simulink model "FCC"  (R2018b)
settings: Solver=FixedStepDiscrete  StartTime=0.0  StopTime=10.0  FixedStep=0.001  RelTol=1e-3  EnableMultiTasking=on
undefined symbols (not defined in the file): Kd, Ki, Kp
libraries: simulink x1
Description:
  | This model represents a flight control system for a helicopter that controls pitch attitude, roll attitude and yaw rate based on pilot inputs from the cyclic and pedals. The flight control computer also closes the loop on three hydrualic actuators and has sensor inputs from three Attitude/Heading Reference Systems.
settings Model: Creator=bpotter  LastModifiedBy=bpotter
settings DataIOCC: LimitDataPoints=on
settings OptimizationCC: BlockReduction=off  DefaultParameterBehavior=Inlined  UseDivisionForNetSlopeComputation=on  InitFltsAndDblsToZero=on  EfficientFloat2IntCast=on  EfficientMapNaN2IntZero=off  LifeSpan=inf  MaxStackSize=inf
settings DebuggingCC: SignalInfNanChecking=error  SignalRangeChecking=error  ReadBeforeWriteMsg=EnableAllAsError  WriteAfterWriteMsg=EnableAllAsError  WriteAfterReadMsg=EnableAllAsError  AlgebraicLoopMsg=error  ArtificialAlgebraicLoopMsg=error  SaveWithDisabledLinksMsg=error  SaveWithParameterizedLinksMsg=error  BlockPriorityViolationMsg=error  SolverPrmCheckMsg=error  InheritedTsInSrcMsg=error  SingleTaskRateTransMsg=error  TasksWithSamePriorityMsg=error  SigSpecEnsureSampleTimeMsg=error  CheckMatrixSingularityMsg=error  IntegerOverflowMsg=error  ParameterUnderflowMsg=error  ParameterPrecisionLossMsg=error  ParameterTunabilityLossMsg=error  UnderSpecifiedDataTypeMsg=error  UnnecessaryDatatypeConvMsg=warning  VectorMatrixConversionMsg=error  SignalLabelMismatchMsg=error  UnconnectedInputMsg=error  UnconnectedOutputMsg=error  UnconnectedLineMsg=error  SFcnCompatibilityMsg=error  UniqueDataStoreMsg=error  BusObjectLabelMismatch=error  RootOutportRequireBusObject=error  AssertControl=DisableAll  AllowSymbolicDim=off  ModelReferenceIOMsg=error  ModelReferenceIOMismatchMessage=error  UnknownTsInhSupMsg=error  ModelReferenceDataLoggingMessage=error  StateNameClashWarn=warning  LibraryContextMissingDiagnostic=none  StrictBusMsg=ErrorOnBusTreatedAsVector  NonBusSignalsTreatedAsBus=error  SFInvalidInputDataAccessInChartInitDiag=error  SFTransitionOutsideNaturalParentDiag=error  SFUnreachableExecutionPathDiag=error  SFUndirectedBroadcastEventsDiag=error  SFTransitionActionBeforeConditionDiag=error  SFExecutionAtInitializationDiag=none  IntegerSaturationMsg=error
settings HardwareCC: ProdBitPerPointer=32  ProdBitPerSizeT=32  ProdBitPerPtrDiffT=32  ProdWordSize=32  ProdHWDeviceType=Intel->x86-32 (Windows32)  TargetIntDivRoundTo=Zero
settings ModelReferenceCC: PropagateSignalLabelsOutOfModel=off
settings SFSimCC: SimUseLocalCustomCode=off  CompileTimeRecursionLimit=0  EnableRuntimeRecursion=off  MATLABDynamicMemAlloc=off
settings RTWCC: SystemTargetFile=ert.tlc  TemplateMakefile=ert_default_tmf  GenerateReport=on  RTWUseLocalCustomCode=off  IncludeHyperlinkInReport=on  LaunchReport=on  PortableWordSizes=on  GenerateTraceInfo=on  GenerateTraceReport=on  GenerateTraceReportSl=on  GenerateTraceReportSf=on  GenerateTraceReportEml=on
settings CodeAppCC: ForceParamTrailComments=on  IgnoreCustomStorageClasses=off  MangleLength=4  StateflowObjectComments=on  ReqsInCode=on
settings ERTTargetCC: TargetLangStandard=C99 (ISO)  UtilityFuncGeneration=Shared location  MultiwordLength=2048  GenerateSampleERTMain=on  IncludeMdlTerminateFcn=off  SuppressErrorStatus=on  SupportAbsoluteTime=off  SupportNonFinite=off  ParenthesesLevel=Maximum  CastingMode=Standards  GenerateSharedConstants=off  ERTCustomFileTemplate=example_file_process.tlc  ERTFilePackagingFormat=Compact  PreserveExpressionOrder=on  PreserveIfCondition=on  ConvertIfToSwitch=off  SuppressUnreachableDefaultCases=off  EnableSignedLeftShifts=off  EnableSignedRightShifts=off
settings ConfigComp: CovMetricSettings=dw  CovHtmlReporting=on  CovSaveCumulativeToWorkspaceVar=on  CovSaveSingleToWorkspaceVar=on  CovExternalEMLEnable=off  CovSFcnEnable=off  PSOpenProjectManager=on  PSResultDir=CodeProver_results_$ModelName$  PSModelRefVerifDepth=All  PSAutoStubLUT=off  DVTestSuiteOptimization=CombinedObjectives (Nonlinear Extended)  DVDetectOutOfBounds=on  DVDesignMinMaxCheck=on

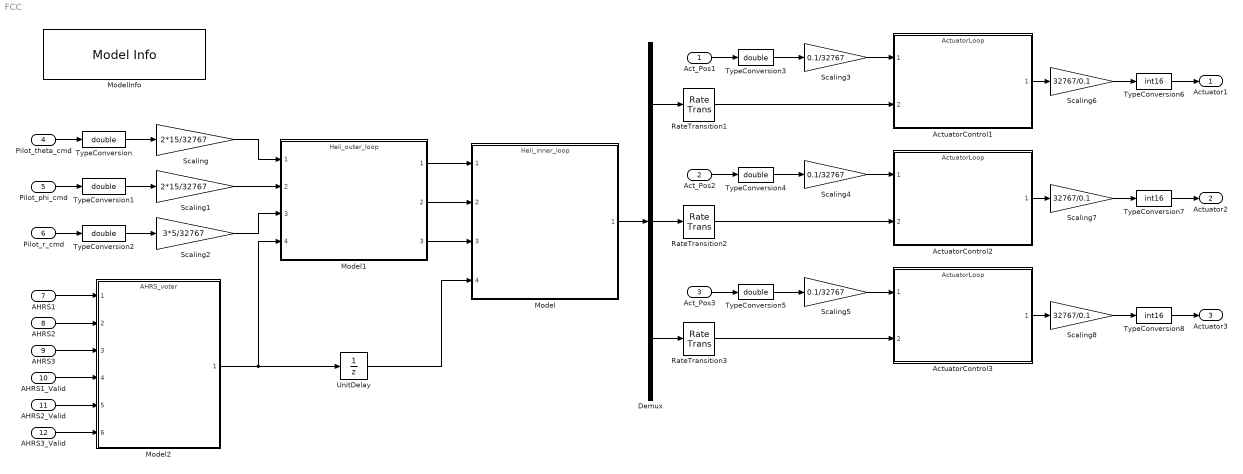
== system FCC ==
  Act_Pos1 : Inport  RequirementInfo={} %GIDa_bd07c6dd_f370_4b97_930d_e4b4981f6696  OutMin=-32768  OutMax=32767  OutDataTypeStr=int16  PortDimensions=1  SampleTime=0.001
  Act_Pos2 : Inport  RequirementInfo={} %GIDa_befe8f2a_df1a_408c_ad43_982e86d61679  Port=2  OutMin=-32768  OutMax=32767  OutDataTypeStr=int16  PortDimensions=1  SampleTime=0.001
  Act_Pos3 : Inport  RequirementInfo={} %GIDa_31a40888_6c46_41b4_95a0_85353469c339  Port=3  OutMin=-32768  OutMax=32767  OutDataTypeStr=int16  PortDimensions=1  SampleTime=0.001
  Pilot_theta_cmd : Inport  RequirementInfo={} %GIDa_db7610c8_fc0b_436a_9176_d063f912f7d4  Port=4  OutMin=-32768  OutMax=32767  OutDataTypeStr=int16  PortDimensions=1  SampleTime=0.01
  Pilot_phi_cmd : Inport  RequirementInfo={} %GIDa_c88793d4_8072_44c9_b7b8_fa9c7a9d095b  Port=5  OutMin=-32768  OutMax=32767  OutDataTypeStr=int16  PortDimensions=1  SampleTime=0.01
  Pilot_r_cmd : Inport  RequirementInfo={} %GIDa_dcbca35e_d37f_4666_ab6e_90461c32e72b  Port=6  OutMin=-32768  OutMax=32767  OutDataTypeStr=int16  PortDimensions=1  SampleTime=0.01
  AHRS1 : Inport  RequirementInfo={} %GIDa_80750aa2_e003_442f_b031_591405abb5b4  Port=7  OutMin=-180  OutMax=180  OutDataTypeStr=double  PortDimensions=5  SampleTime=0.01
  AHRS2 : Inport  RequirementInfo={} %GIDa_426ecfe9_991d_4f5f_80a1_3ebd9c43cb2d  Port=8  OutMin=-180  OutMax=180  OutDataTypeStr=double  PortDimensions=5  SampleTime=0.01
  AHRS3 : Inport  RequirementInfo={} %GIDa_78c653e8_6a57_498e_82a6_5c1330482b46  Port=9  OutMin=-180  OutMax=180  OutDataTypeStr=double  PortDimensions=5  SampleTime=0.01
  AHRS1_Valid : Inport  RequirementInfo={} %GIDa_98b30cb9_b983_4ea0_884e_7d00cc40e0ae  Port=10  OutMin=0  OutMax=1  OutDataTypeStr=boolean  PortDimensions=1  SampleTime=0.01
  AHRS2_Valid : Inport  RequirementInfo={} %GIDa_97bebaab_bb97_4960_9c93_3ab597d65b2c  Port=11  OutMin=0  OutMax=1  OutDataTypeStr=boolean  PortDimensions=1  SampleTime=0.01
  AHRS3_Valid : Inport  RequirementInfo={} %GIDa_19fd269e_922e_4b90_a0a1_f582c1a1233f  Port=12  OutMin=0  OutMax=1  OutDataTypeStr=boolean  PortDimensions=1  SampleTime=0.01
  ActuatorControl1 : ModelReference  RequirementInfo={} %GIDa_286e3d14_20d8_4bab_aa60_69e0b735c692  ModelNameDialog=ActuatorLoop  ParameterArgumentNames=Kp,Kd,Ki  ParameterArgumentValues=0.3,0.02,0.12  UsingDefaultArgumentValue=0,0,0  SimulationMode=Normal  ModelReferenceVersion=1.40
  ActuatorControl2 : ModelReference  RequirementInfo={} %GIDa_6f1d74b9_a492_4876_bea7_840580edc6b2  ModelNameDialog=ActuatorLoop  ParameterArgumentNames=Kp,Kd,Ki  ParameterArgumentValues=0.3,0.02,0.12  UsingDefaultArgumentValue=0,0,0  SimulationMode=Normal  ModelReferenceVersion=1.40
  ActuatorControl3 : ModelReference  RequirementInfo={} %GIDa_5780c5a5_fbb9_4ac7_8106_2a6374d1c9b6  ModelNameDialog=ActuatorLoop  ParameterArgumentNames=Kp,Kd,Ki  ParameterArgumentValues=0.3,0.02,0.12  UsingDefaultArgumentValue=0,0,0  SimulationMode=Normal  ModelReferenceVersion=1.40
  Demux : Demux  Outputs=3
  Model : ModelReference  RequirementInfo={} %GIDa_9f86ca98_8be5_4c76_b7e2_fad36800e068  ModelNameDialog=Heli_inner_loop  SimulationMode=Normal  ModelReferenceVersion=1.29
  Model1 : ModelReference  RequirementInfo={} %GIDa_9b6918d6_c850_456e_b2c9_5fe3f7942cab  ModelNameDialog=Heli_outer_loop  SimulationMode=Normal  ModelReferenceVersion=1.27
  Model2 : ModelReference  RequirementInfo={} %GIDa_45ae46d8_e7b6_4c79_9f98_fde151ca045a  ModelNameDialog=AHRS_voter  SimulationMode=Normal  ModelReferenceVersion=1.56
  ModelInfo : simulink/Model-Wide Utilities/Model Info  Frame=on  DisplayStringWithTags=|  HorizontalTextAlignment=Center  LeftAlignmentValue=0.5
      | Model Name: %<ModelName>
      | Model Version: %<ModelVersion>
      | Last Modified: %<LastModificationDate>
      | 
      | Copyright 2016 The MathWorks, Inc.
  RateTransition1 : RateTransition  OutPortSampleTime=0.001
  RateTransition2 : RateTransition  OutPortSampleTime=0.001
  RateTransition3 : RateTransition  OutPortSampleTime=0.001
  Scaling : Gain  RequirementInfo={} %GIDa_1ef55a73_43a4_45d8_95fb_e076cecdcdfb  Gain=2*15/32767
  Scaling1 : Gain  RequirementInfo={} %GIDa_7c0c4402_eed7_48e8_afe7_4e3c25c20a7a  Gain=2*15/32767
  Scaling2 : Gain  RequirementInfo={} %GIDa_c573d4b7_5d38_46e9_91de_b74deab4371c  Gain=3*5/32767
  Scaling3 : Gain  RequirementInfo={} %GIDa_7165c314_723d_4c07_8145_b8a5caf68d15  Gain=0.1/32767
  Scaling4 : Gain  RequirementInfo={} %GIDa_e7d939dc_4756_4c7f_b09b_37bf3b41d91a  Gain=0.1/32767
  Scaling5 : Gain  RequirementInfo={} %GIDa_feb82ae6_ad6e_4307_be71_c8336adce306  Gain=0.1/32767
  Scaling6 : Gain  RequirementInfo={} %GIDa_7472457d_0776_496d_982d_888a9d0ccd31  Gain=32767/0.1  SaturateOnIntegerOverflow=on  OutDataTypeStr=Inherit: Same as input
  Scaling7 : Gain  RequirementInfo={} %GIDa_27270bf9_988e_4404_bcbc_b8b952500a10  Gain=32767/0.1  SaturateOnIntegerOverflow=on  OutDataTypeStr=Inherit: Same as input
  Scaling8 : Gain  RequirementInfo={} %GIDa_610bafad_081e_4b34_b128_56987096ac68  Gain=32767/0.1  SaturateOnIntegerOverflow=on  OutDataTypeStr=Inherit: Same as input
  TypeConversion : DataTypeConversion  RequirementInfo={} %GIDa_507dfc48_2783_4f54_bcc8_b8696a72db7e  OutDataTypeStr=double
  TypeConversion1 : DataTypeConversion  RequirementInfo={} %GIDa_a28ee961_0826_464b_952a_7525a850e69d  OutDataTypeStr=double
  TypeConversion2 : DataTypeConversion  RequirementInfo={} %GIDa_fd029ccd_092a_44ae_ba63_7ba73a38dd29  OutDataTypeStr=double
  TypeConversion3 : DataTypeConversion  RequirementInfo={} %GIDa_1949c14f_f47a_4a2c_b83b_c5a889847ffe  OutDataTypeStr=double
  TypeConversion4 : DataTypeConversion  RequirementInfo={} %GIDa_29dd9675_a919_4bb5_a5f8_82f3a5941f34  OutDataTypeStr=double
  TypeConversion5 : DataTypeConversion  RequirementInfo={} %GIDa_0de29fa2_9bc9_4717_a2b2_9bc25147b395  OutDataTypeStr=double
  TypeConversion6 : DataTypeConversion  RequirementInfo={} %GIDa_6ab4c5ff_fe2f_4ca3_924f_fd1b53f5822d  OutDataTypeStr=int16
  TypeConversion7 : DataTypeConversion  RequirementInfo={} %GIDa_fe351f61_f1d0_4404_aa3c_5114a8d4af07  OutDataTypeStr=int16
  TypeConversion8 : DataTypeConversion  RequirementInfo={} %GIDa_5d4fc6d9_c4e4_4413_b6aa_2af104ad7bd2  OutDataTypeStr=int16
  UnitDelay : UnitDelay  SampleTime=-1
  Actuator1 : Outport  RequirementInfo={} %GIDa_0e27a381_736b_4604_a443_1ce3b6bc89bb
  Actuator2 : Outport  RequirementInfo={} %GIDa_ad165c3e_4ab6_4671_aa0b_225d448592bb  Port=2
  Actuator3 : Outport  RequirementInfo={} %GIDa_f2f33165_edb5_46cb_9250_52960ae67539  Port=3
  wires:
  ActuatorControl1/1 -> Scaling6/1
  ActuatorControl2/1 -> Scaling7/1
  ActuatorControl3/1 -> Scaling8/1
  RateTransition1/1 -> ActuatorControl1/2
  RateTransition2/1 -> ActuatorControl2/2
  RateTransition3/1 -> ActuatorControl3/2
  AHRS2/1 -> Model2/2
  AHRS3/1 -> Model2/3
  Demux/1 -> RateTransition1/1
  Demux/2 -> RateTransition2/1
  Demux/3 -> RateTransition3/1
  Model/1 -> Demux/1
  Model1/1 -> Model/1
  Model1/2 -> Model/2
  Model1/3 -> Model/3
  AHRS1/1 -> Model2/1
  Model2/1 -> Model1/4, UnitDelay/1
  AHRS1_Valid/1 -> Model2/4
  AHRS2_Valid/1 -> Model2/5
  AHRS3_Valid/1 -> Model2/6
  TypeConversion/1 -> Scaling/1
  Pilot_theta_cmd/1 -> TypeConversion/1
  Scaling/1 -> Model1/1
  TypeConversion1/1 -> Scaling1/1
  Pilot_phi_cmd/1 -> TypeConversion1/1
  Scaling1/1 -> Model1/2
  Pilot_r_cmd/1 -> TypeConversion2/1
  TypeConversion2/1 -> Scaling2/1
  Scaling2/1 -> Model1/3
  TypeConversion3/1 -> Scaling3/1
  Act_Pos1/1 -> TypeConversion3/1
  Scaling3/1 -> ActuatorControl1/1
  TypeConversion4/1 -> Scaling4/1
  TypeConversion5/1 -> Scaling5/1
  Act_Pos2/1 -> TypeConversion4/1
  Scaling4/1 -> ActuatorControl2/1
  Act_Pos3/1 -> TypeConversion5/1
  Scaling5/1 -> ActuatorControl3/1
  Scaling6/1 -> TypeConversion6/1
  Scaling7/1 -> TypeConversion7/1
  Scaling8/1 -> TypeConversion8/1
  TypeConversion6/1 -> Actuator1/1
  TypeConversion7/1 -> Actuator2/1
  TypeConversion8/1 -> Actuator3/1
  UnitDelay/1 -> Model/4
